simulink model "dsp_audio_player_v1"  (R2020b)
settings: Solver=FixedStepDiscrete  StartTime=0.0  StopTime=Inf  RelTol=1e-3  EnableMultiTasking=on
undefined symbols (not defined in the file or in its folder): A, data, GPTRIP1SEL, GPTRIP2SEL, TZ1, TZ2
libraries: simulink x8, idelinklib_common x3, c280xlib x3, c2837xDlib x2, dspxfrm3 x2, c2000lib x1, c2802xlib x1
settings Model: ExtModeTrigDuration=8  Creator=adria  LastModifiedBy=tyler
settings OptimizationCC: DefaultUnderspecifiedDataType=single  EnhancedBackFolding=on  PassReuseOutputArgsAs=Individual arguments  MaxStackSize=1024  OptimizeBlockOrder=speed  DifferentSizesBufferReuse=on  OptimizationCustomize=off  DenormalBehavior=FlushToZero  EfficientTunableParamExpr=on
settings DebuggingCC: MultiTaskDSMMsg=none  ParameterTunabilityLossMsg=error
settings HardwareCC: ProdBitPerChar=16  ProdBitPerInt=16  ProdBitPerPointer=32  ProdBitPerSizeT=32  ProdBitPerPtrDiffT=32  ProdLargestAtomicInteger=Integer  ProdLargestAtomicFloat=None  ProdWordSize=16  ProdLongLongMode=on  ProdHWDeviceType=Texas Instruments->C2000
settings SFSimCC: MATLABDynamicMemAlloc=off
settings RTWCC: Description=Embedded Coder  SystemTargetFile=ert.tlc  HardwareBoard=TI Delfino F28379D LaunchPad  TemplateMakefile=ert_default_tmf  GenerateReport=on  Toolchain=Texas Instruments Code Composer Studio (C2000)  LaunchReport=on
settings CodeAppCC: ForceParamTrailComments=on  IgnoreCustomStorageClasses=off  OperatorAnnotations=on  SimulinkDataObjDesc=on  SFDataObjDesc=on  InsertBlockDesc=on
settings ERTTargetCC: CodeReplacementLibrary=TI C28x  ExtModeTransport=3  ExtModeStaticAllocSize=10000

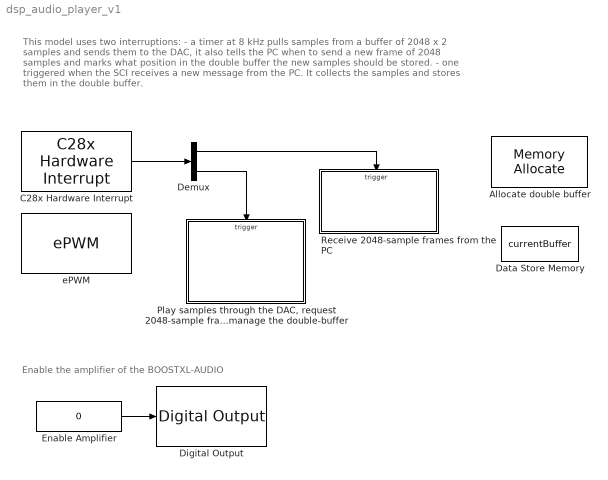
== system dsp_audio_player_v1 ==
  note: This model uses two interruptions:
      | - a timer at 8 kHz pulls samples from a buffer of 2048 x 2 samples and sends them to the DAC, it also tells the PC when to send a new frame of 2048 samples and marks what position in the double buffer the new samples should be stored.
      | - one triggered when the SCI receives a new message from the PC. It collects the samples and stores them in the double buffer.
  note: Enable the amplifier of the BOOSTXL-AUDIO
  Allocate double buffer : idelinklib_common/Memory Allocate  variableName=doubleBuffer  alignThisVariable=off  memoryAlignmentBoundary=4  dataType=uint16  specifyQualifier=off  typeQualifier=volatile  dataDimension=2^12  specifyMemorySection=off  memorySection=mySEC1  bindMemorySection=off  sectionStartAddress=hex2dec('8000')  initializeMemory=on  initialValue=zeros(1,(2^12))
      settings: SourceProductBaseCode=ME
  C28x Hardware Interrupt : c2000lib/Scheduling/C28x Hardware Interrupt  irqnumbers=[9 3]  pienumbers=[1 1]  irqpriorities=[50 30]  irqpreempts=[0 0]  showinput=off  dspchiptype=C280X
      settings: SourceProductName=Embedded Coder Support Package for Texas Instruments C2000 Processors
  Data Store Memory : DataStoreMemory  DataStoreName=currentBuffer  ReadBeforeWriteMsg=warning  WriteAfterWriteMsg=warning  WriteAfterReadMsg=warning  ShowAdditionalParam=off  OutDataTypeStr=uint16
  Demux : Demux  Outputs=2
  Digital Output : c2837xDlib/Digital Output  GPIO_Number=GPIO24~GPIO31  GPIO_Bit0=off  GPIO_BIT0_Toggle=off  GPIO_Bit1=off  GPIO_BIT1_Toggle=off  GPIO_Bit2=on  GPIO_BIT2_Toggle=off  GPIO_Bit3=off  GPIO_BIT3_Toggle=off  GPIO_Bit4=off  GPIO_BIT4_Toggle=off  GPIO_Bit5=off  GPIO_BIT5_Toggle=off  GPIO_Bit6=off  GPIO_BIT6_Toggle=off  GPIO_Bit7=off  GPIO_BIT7_Toggle=off
      settings: SourceProductBaseCode=TIC2000
  Enable Amplifier : Constant  Value=0
  "Play samples through the DAC, request 2048-sample frames from the PC, manage the double-buffer" : Subsystem
  Receive 2048-sample frames from the PC : Subsystem
  ePWM : c2802xlib/ePWM  PwmType=C2000_Type4  useModule=ePWM1  ePWMxLINKTBPRD=Not Linked  periodUnits=Seconds  timerSource=Specify via dialog  timerPeriod_clk=1000  timerPeriod_sec=1/8000  tbshadow=Counter equals to zero  countingMode=Up  phaseActiveEnable=Disable  phaseDirection=Count down after sync  phaseActive=0  synchronizationEnable=off  dcaevt1Sync=off  dcbevt1Sync=off  synchronizationOption=Disable  perSynchronizationOption=Counter equals to period (CTR=PRD)  clockPrescale=1  HSclockPrescale=1  enswap=off  ePWMxAStatus=on  ePWMxAactionLogic1=Do nothing  ePWMxAactionLogic2=Do nothing  ePWMxAactionLogic3=Do nothing  ePWMxAactionLogic4=Set  ePWMxAactionLogic5=Do nothing  ePWMxAactionLogic6=Do nothing  ePWMxACSFenable=off  ePWMxACSFvalue=Forcing disable  ePWMxASFreload=Zero  ePWMxBStatus=off  ePWMxBactionLogic1=Set  ePWMxBactionLogic2=Clear  ePWMxBactionLogic3=Do nothing  ePWMxBactionLogic4=Do nothing  ePWMxBactionLogic5=Clear  ePWMxBactionLogic6=Set  ePWMxBCSFenable=off  ePWMxBCSFvalue=Forcing disable  ePWMxBSFreload=Zero  ePWNxBOutWay=off  ePWMxLINKCMPA=Not Linked  CMPAUnits=Percentages  CMPASource=Specify via dialog  CMPAValue_per=50  CMPAValue_clk=50  enCMPAshadow=Counter equals to zero (CTR=Zero)  ePWMxLINKCMPB=Not Linked  CMPBUnits=Clock cycles  CMPBSource=Specify via dialog  CMPBValue_per=50  CMPBValue_clk=32000  enCMPBshadow=Counter equals to zero (CTR=Zero)  ePWMxLINKCMPC=Not Linked  CMPCUnits=Clock cycles  CMPCSource=Specify via dialog  CMPCValue_per=50  CMPCValue_clk=32000  enCMPCshadow=Counter equals to zero (CTR=Zero)  ePWMxLINKCMPD=Not Linked  CMPDUnits=Clock cycles  CMPDSource=Specify via dialog  CMPDValue_per=50  CMPDValue_clk=32000  enCMPDshadow=Counter equals to zero (CTR=Zero)  enableDBePWMxA=off  enableDBePWMxB=off  enhalfcycle=off  DBpolarity=Active high (AH)  DBedgeDelay=Positive  DBSource_ePWMxA=ePWMxA  DBSource_ePWMxB=ePWMxA  DBPeriodUnits=Clock cycles  DBperiodSource=Specify via dialog  REDperiod=0  FEDperiod=0  REDperiod_sec=0  FEDperiod_sec=0  LoadModeDBRED=Immediate without using shadow  LoadModeDBFED=Immediate without using shadow  adcstartModuleA=off  adcrequestEventA=First event  adcstartEventA=Digital Compare Module A Event 1 start of conversion (DCAEVT1.soc)  adcstartEventA_type2=Digital Compare Module A Event 1 start of conversion (DCAEVT1.soc)  adcstartModuleB=off  adcrequestEventB=First event  adcstartEventB=Counter equals to zero (CTR=Zero)  adcstartEventB_type2=Counter equals to zero (CTR=Zero)  intEn=on  intPrd=First event  intSel=Counter equals to zero (CTR=Zero)  intSel_type2=Counter equals to zero (CTR=Zero)  hrpe=off  enHRPWM=off  HRPWM_LoadMode=Counter equals to period (CTR=PRD)  HRPWM_CTLMode=Duty or Period control mode  HRPWM_EDGMode=Both edge  hrpeb=off  enHRPWMB=off  HRPWM_LoadModeB=Counter equals to zero (CTR=ZERO)  HRPWM_CTLModeB=Duty or Period control mode  HRPWM_EDGModeB=Both edge  enHRDBRED=off  enHRDBFED=off  enSFO=on  enautoconv=on  chopperEnable=off  chopperFrequency=1  chopperFirstwidth=1  chopperDuty=12.5%  tripZonesource=Specify via dialog  tzselOSHT1=off  tzselOSHT2=off  tzselOSHT3=off  tzselOSHDCAEV1=off  tzselOSHDCBEV1=off  tzselCBC1=off  tzselCBC2=off  tzselCBC3=off  tzselCBCDCAEV2=off  tzselCBCDCBEV2=off  tzselOSHT4=off  tzselOSHT5=off  tzselOSHT6=off  tzselCBC4=off  tzselCBC5=off  tzselCBC6=off  enTzOstIntr=off  enTzCbcIntr=off  enTzDCAEVT1Intr=off  enTzDCAEVT2Intr=off  enTzDCBEVT1Intr=off  enTzDCBEVT2Intr=off  ePWMxAforced=No action  ePWMxBforced=No action  DCAEVT1forced=No action  DCBEVT1forced=No action  DCAEVT2forced=No action  DCBEVT2forced=No action  dcah=Trip Zone 1 input (TZ1)  dcal=Trip Zone 2 input (TZ2)  dcbh=Trip Zone 1 input (TZ1)  dcbl=Trip Zone 2 input (TZ2)  dcah_type2=GPTRIP1SEL/(TZ1)  dcal_type2=GPTRIP2SEL/(TZ2)  dcbh_type2=GPTRIP1SEL/(TZ1)  dcbl_type2=GPTRIP2SEL/(TZ2)  gendcaevt1=Event disabled  gendcaevt2=Event disabled  gendcbevt1=Event disabled  gendcbevt2=Event disabled  dcaevt1src=DCAEVT1 with sync  dcaevt2src=DCAEVT2 with sync  dcbevt1src=DCBEVT1 with sync  dcbevt2src=DCBEVT2 with sync  pulsesel=Counter equals to zero (CTR=Zero)  blankinv=off  blankoffset=0  blankwidth=0  evsrcsel=Filtered version of DCAEVT1 (DCAEVT1FILT)  encape=off
      settings: SourceProductName=Embedded Coder Support Package for Texas Instruments C2000 Processors
  wires:
  C28x Hardware Interrupt/1 -> Demux/1
  Demux/1 -> Receive 2048-sample frames from the PC/Trigger
  Demux/2 -> "Play samples through the DAC, request 2048-sample frames from the PC, manage the double-buffer"/Trigger
  Enable Amplifier/1 -> Digital Output/1

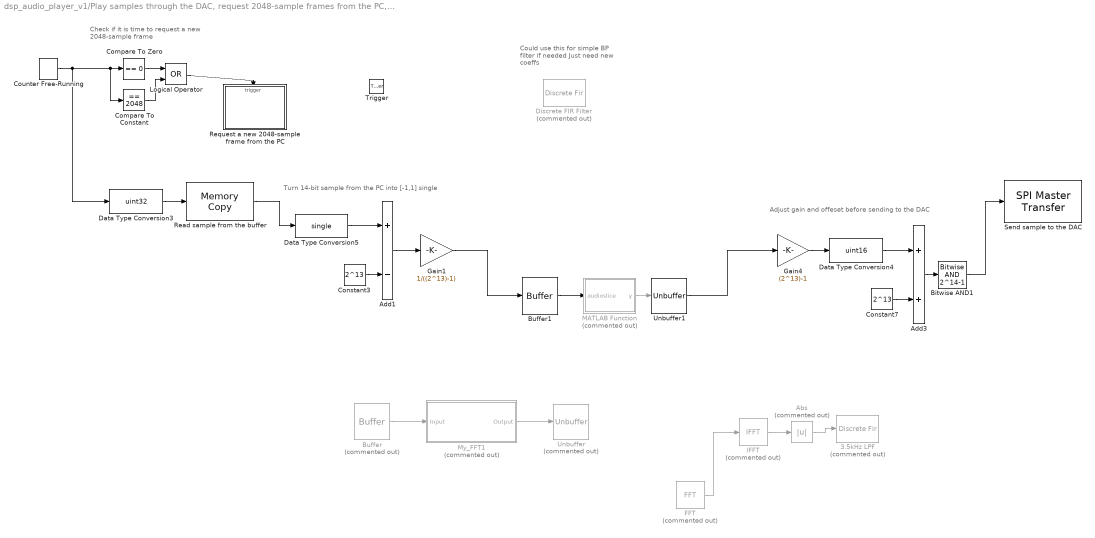
== system dsp_audio_player_v1/Play samples through the DAC, request 2048-sample frames from the PC, manage the double-buffer ==
  note: Could use this for
      | simple BP filter if needed
      | Just need new coeffs
  note: Turn 14-bit sample from the PC into [-1,1] single
  note: Adjust gain and offeset before sending to the DAC
  note: Check if it is time to request
      | a new 2048-sample frame
  Trigger : TriggerPort  TriggerType=function-call  VariantControl=Variant  PortDimensions=1
  3.5kHz LPF : DiscreteFir  Commented=on  Coefficients=[-0.000400517864648427,-0.00597270631126555,-0.00588600875883281,0.00305220673006901,0.00340984153034900,-0.00584791328673356,-0.000942482039609760,0.00831300701616265,-0.00350292218202603,-0.00903364920390202,0.00977259721520285,0.00633489663026340,-0.0164864938688951,0.00112630892188619,0.0210980048311115,-0.0137454614242812,-0.0201583607432012,0.0305294671131217,0.00951594876559339,-0.0490740358099981,0.0166730488518273,0.0660460111384453,-0.0743550579470649,-0.0779651266053814,0.307083541990112,0.582258998534139,0.307083541990112,-0.0779651266053814,-0.0743550579470649,0.0660460111384453,0.0166730488518273,-0.0490740358099981,0.00951594876559339,0.0305294671131217,-0.0201583607432012,-0.0137454614242812,0.0210980048311115,0.00112630892188619,-0.0164864938688951,0.00633489663026340,0.00977259721520285,-0.00903364920390202,-0.00350292218202603,0.00831300701616265,-0.000942482039609760,-0.00584791328673356,0.00340984153034900,0.00305220673006901,-0.00588600875883281,-0.00597270631126555,-0.000400517864648427]
  Abs : Abs  Commented=on
  Add1 : Sum  Inputs=+-
  Add3 : Sum
  Bitwise AND1 : simulink/Logic and Bit Operations/Bitwise Operator  logicop=AND  UseBitMask=on  BitMask=2^14-1  BitMaskRealWorld=Stored Integer
  Buffer : Buffer  Commented=on  N=16  V=15  OutputFrames=off
  Buffer1 : Buffer  N=2048  V=2047  OutputFrames=off
  Compare To Constant : simulink/Logic and Bit Operations/Compare To Constant  relop===  const=2048  OutDataTypeStr=boolean
  Compare To Zero : simulink/Logic and Bit Operations/Compare To Zero  relop===  OutDataTypeStr=boolean
  Constant3 : Constant  Value=2^13  OutDataTypeStr=single
  Constant7 : Constant  Value=2^13  OutDataTypeStr=uint16
  Counter Free-Running : simulink/Sources/Counter Free-Running  NumBits=12  tsamp=-1
  Data Type Conversion3 : DataTypeConversion  OutDataTypeStr=uint32
  Data Type Conversion4 : DataTypeConversion  OutDataTypeStr=uint16
  Data Type Conversion5 : DataTypeConversion  OutDataTypeStr=single
  Discrete FIR Filter : DiscreteFir  Commented=on  Coefficients="[-0.000810102636137497\t-0.000392374131282647\t-4.06563948247084e-05\t0.000767451730429069\t0.00204102792071147\t0.00363434793640914\t0.00522314138161502\t0.00632871351818929\t0.00639886630822526\t0.00494089174170842\t0.00168166719513044\t-0.00327772717740523\t-0.00935730346277267\t-0.0154836748342822\t-0.0201875759335370\t-0.0218139413210731\t-0.0188190039298270\t-0.0101023307256181\t0.00469465139069746\t0.0249940309565858\t0.0492440262935009\t0.0750604816349442\t0.0995424525458068\t0.119710733564489\t0.132986042515205\t0.137615586465308\t0.132986042515205\t0.119710733564489\t0.0995424525458068\t0.0750604816349442\t0.0492440262935009\t0.0249940309565858\t0.00469465139069746\t-0.0101023307256181\t-0.0188190039298270\t-0.0218139413210731\t-0.0201875759335370\t-0.0154836748342822\t-0.00935730346277267\t-0.00327772717740523\t0.00168166719513044\t0.00494089174170842\t0.00639886630822526\t0.00632871351818929\t0.00522314138161502\t0.00363434793640914\t0.00204102792071147\t0.000767451730429069\t-4.06563948247084e-05\t-0.000392374131282647\t-0.000810102636137497]"
  FFT : dspxfrm3/FFT  Commented=on  FFTImplementation=Auto  CompMethod=Table lookup  TableOpt=NEW  TableOptActive=Speed  BitRevOrder=off  Normalize=off  InheritFFTLength=on  FFTLength=64  WrapInput=on  roundingMode=Floor  overflowMode=off  firstCoeffDataTypeStr=Inherit: Same word length as input  firstCoeffLastDataTypeStr=Inherit: Same word length as input  outputMin=[]  outputMax=[]
  Gain1 : Gain  Gain=1/((2^13)-1)
  Gain4 : Gain  Gain=(2^13)-1
  IFFT : dspxfrm3/IFFT  Commented=on  FFTImplementation=Auto  CompMethod=Table lookup  TableOpt=NEW  TableOptActive=Speed  BitRevOrder=off  cs_in=off  Normalize=on  InheritFFTLength=on  FFTLength=64  WrapInput=on  mode=Complex  outSamplingMode=Sample based  roundingMode=Floor  overflowMode=off  firstCoeffDataTypeStr=Inherit: Same word length as input  firstCoeffLastDataTypeStr=Inherit: Same word length as input  outputMin=[]  outputMax=[]
  Logical Operator : Logic  Operator=OR  AllPortsSameDT=off  OutDataTypeStr=boolean
  MATLAB Function : MATLAB Function  Commented=on  TreatAsAtomicUnit=on
  My_FFT1 : Subsystem  Commented=on
  Read sample from the buffer : idelinklib_common/Memory Copy  copyFrom=Specified source code symbol  copyFromAddressSource=Specify via dialog  copyFromAddress=hex2dec('00001000')  copyFromSrcCode=doubleBuffer  dataTypeFrom=uint16  dataDimensionFrom=1  useOffsetFrom=on  offsetFromSrc=Input port  offsetFrom=0  strideFrom=1  copyTo=Output port  copyToAddressSource=Specify via dialog  copyToAddress=hex2dec('00002000')  copyToSrcCode=myVariable  dataTypeTo=uint16  useOffsetTo=off  offsetToSrc=Input port  offsetTo=0  strideTo=1  sampleTime=-1  useInitValue=off  initValueSrc=Specify constant value  initValue=1  initValueSrcCode=myInitValueVariable  useAsMask=off  maskOperator=bitwise AND  useTermValue=off  termValue=1  isRealtimeEnabled=off  emitCCBeforeWrite=off  CCBeforeWrite=/* Custom Code Before Write*/  emitCCAfterWrite=off  CCAfterWrite=/* Custom Code After Write*/  useDMACopy=off  enableBlockingMode=off
      settings: SourceProductBaseCode=ME
  Request a new 2048-sample frame from the PC : Subsystem
  Send sample to the DAC : c280xlib/SPI Master Transfer  SPISelect=SPI_B  ClockPolarity=Rising_edge  ClockPhase=Delay_half_cycle  SPIModule=uint32(0)  Mode=Master  BusSpeed=uint32(1000000)  FirstBitToTransfer=Most significant bit (MSB)  ClockMode=0  BlockFunction=Transfer  EnableRegisterAddress=off  RegisterAddress=0  OutputDataType=int8  OutputDataLength=1  DataBits=16  UseCustomSSPin=Explicit GPIO calls  ActiveLowSSPin=Active low  Pin=27
      settings: SourceProductName=Embedded Coder Support Package for Texas Instruments C2000 Processors
  Unbuffer : Unbuffer  Commented=on
  Unbuffer1 : Unbuffer
  wires:
  Data Type Conversion3/1 -> Read sample from the buffer/1
  Compare To Zero/1 -> Logical Operator/1
  Compare To Constant/1 -> Logical Operator/2
  Logical Operator/1 -> Request a new 2048-sample frame from the PC/Trigger
  Counter Free-Running/1 -> Compare To Constant/1, Compare To Zero/1, Data Type Conversion3/1
  Add3/1 -> Bitwise AND1/1
  Gain4/1 -> Data Type Conversion4/1
  Constant7/1 -> Add3/2
  Data Type Conversion4/1 -> Add3/1
  Constant3/1 -> Add1/2
  Data Type Conversion5/1 -> Add1/1
  Add1/1 -> Gain1/1
  Read sample from the buffer/1 -> Data Type Conversion5/1
  Bitwise AND1/1 -> Send sample to the DAC/1
  My_FFT1/1(Output) -> Unbuffer/1
  Buffer/1 -> My_FFT1/1(Input)
  Gain1/1 -> Buffer1/1
  Abs/1 -> 3.5kHz LPF/1
  FFT/1 -> IFFT/1
  IFFT/1 -> Abs/1
  Buffer1/1 -> MATLAB Function/1(audioslice)
  MATLAB Function/1(y) -> Unbuffer1/1
  Unbuffer1/1 -> Gain4/1

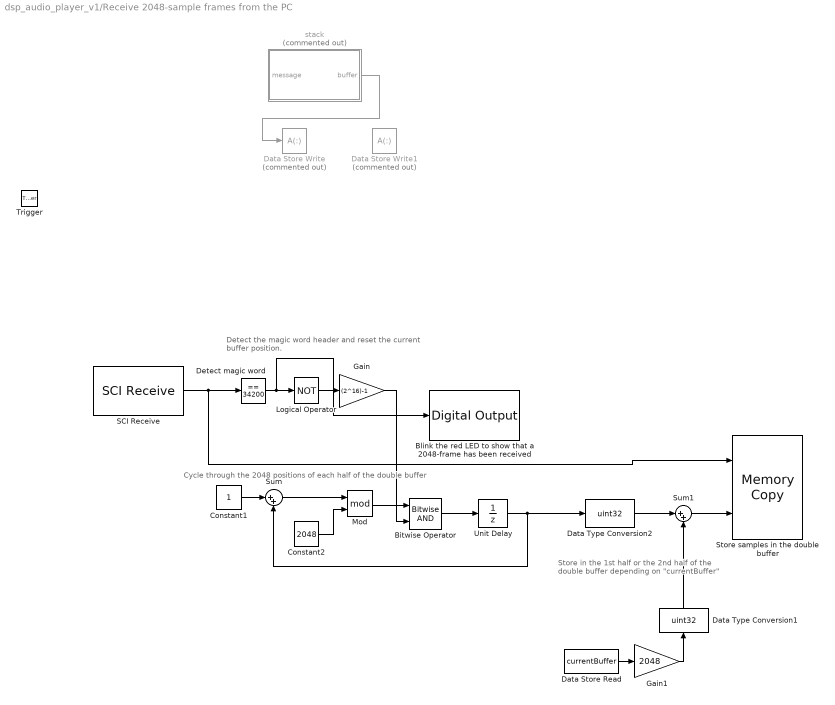
== system dsp_audio_player_v1/Receive 2048-sample frames from the PC ==
  note: Store in the 1st half or the 2nd half
      | of the double buffer depending on
      | "currentBuffer"
  note: Cycle through the 2048 positions of each half of the double buffer
  note: Detect the magic word header and
      | reset the current buffer position.
  Trigger : TriggerPort  TriggerType=function-call  VariantControl=Variant  PortDimensions=1
  Bitwise Operator : simulink/Logic and Bit Operations/Bitwise Operator  logicop=AND  UseBitMask=off  NumInputPorts=2  BitMask=bin2dec('11011001')  BitMaskRealWorld=Stored Integer
  Blink the red LED to show that a 2048-frame has been received : c2837xDlib/Digital Output  GPIO_Number=GPIO32~GPIO39  GPIO_Bit0=off  GPIO_BIT0_Toggle=off  GPIO_Bit1=off  GPIO_BIT1_Toggle=off  GPIO_Bit2=on  GPIO_BIT2_Toggle=on  GPIO_Bit3=off  GPIO_BIT3_Toggle=off  GPIO_Bit4=off  GPIO_BIT4_Toggle=on  GPIO_Bit5=off  GPIO_BIT5_Toggle=off  GPIO_Bit6=off  GPIO_BIT6_Toggle=off  GPIO_Bit7=off  GPIO_BIT7_Toggle=off
      settings: SourceProductBaseCode=TIC2000
  Constant1 : Constant  OutDataTypeStr=uint16  SampleTime=-1
  Constant2 : Constant  Value=2048  OutDataTypeStr=uint16  SampleTime=-1
  Data Store Read : DataStoreRead  DataStoreName=currentBuffer
  Data Store Write : DataStoreWrite  Commented=on  DataStoreElements=A(:)
  Data Store Write1 : DataStoreWrite  Commented=on  DataStoreElements=A(:)
  Data Type Conversion1 : DataTypeConversion  OutDataTypeStr=uint32
  Data Type Conversion2 : DataTypeConversion  OutDataTypeStr=uint32
  Detect magic word : simulink/Logic and Bit Operations/Compare To Constant  relop===  const=34200  OutDataTypeStr=boolean
  Gain : Gain  Gain=(2^16)-1  OutDataTypeStr=uint16
  Gain1 : Gain  Gain=2048  OutDataTypeStr=uint16
  Logical Operator : Logic  Operator=NOT  AllPortsSameDT=off  OutDataTypeStr=boolean
  Mod : Math  Operator=mod  SaturateOnIntegerOverflow=on
  SCI Receive : c280xlib/SCI Receive  sciModule=A  dataHead=''  dataTail=''  dataType=uint16  dataDim=1  initValue=0  errOption=Output the last received value  errValue=0  sampleTime=-1  outputStatus=off  postInterrupt=on  numFifo=2
      settings: SourceProductName=Embedded Coder Support Package for Texas Instruments C2000 Processors
  Store samples in the double buffer : idelinklib_common/Memory Copy  copyFrom=Input port  copyFromAddressSource=Specify via dialog  copyFromAddress=hex2dec('00001000')  copyFromSrcCode=myVariableSrc  dataTypeFrom=uint16  dataDimensionFrom=1  useOffsetFrom=off  offsetFromSrc=Specify via dialog  offsetFrom=0  strideFrom=1  copyTo=Specified source code symbol  copyToAddressSource=Specify via dialog  copyToAddress=hex2dec('00002000')  copyToSrcCode=doubleBuffer  dataTypeTo=uint16  useOffsetTo=on  offsetToSrc=Input port  offsetTo=0  strideTo=1  sampleTime=-1  useInitValue=off  initValueSrc=Specify constant value  initValue=1  initValueSrcCode=myInitValueVariable  useAsMask=off  maskOperator=bitwise AND  useTermValue=off  termValue=1  isRealtimeEnabled=off  emitCCBeforeWrite=off  CCBeforeWrite=/* Custom Code Before Write*/  emitCCAfterWrite=off  CCAfterWrite=/* Custom Code After Write*/  useDMACopy=off  enableBlockingMode=off
      settings: SourceProductBaseCode=ME
  Sum : Sum  Inputs=|++
  Sum1 : Sum  Inputs=|++
  Unit Delay : UnitDelay  SampleTime=-1  HasFrameUpgradeWarning=on
  stack : Subsystem  Commented=on
  wires:
  stack/1(buffer) -> Data Store Write/1
  Unit Delay/1 -> Data Type Conversion2/1, Sum/2
  Detect magic word/1 -> Logical Operator/1, Blink the red LED to show that a 2048-frame has been received/1
  Constant1/1 -> Sum/1
  Sum/1 -> Mod/1
  Constant2/1 -> Mod/2
  SCI Receive/1 -> Detect magic word/1, Store samples in the double buffer/1
  Mod/1 -> Bitwise Operator/1
  Gain/1 -> Bitwise Operator/2
  Bitwise Operator/1 -> Unit Delay/1
  Data Store Read/1 -> Gain1/1
  Data Type Conversion2/1 -> Sum1/1
  Sum1/1 -> Store samples in the double buffer/2
  Gain1/1 -> Data Type Conversion1/1
  Data Type Conversion1/1 -> Sum1/2
  Logical Operator/1 -> Gain/1

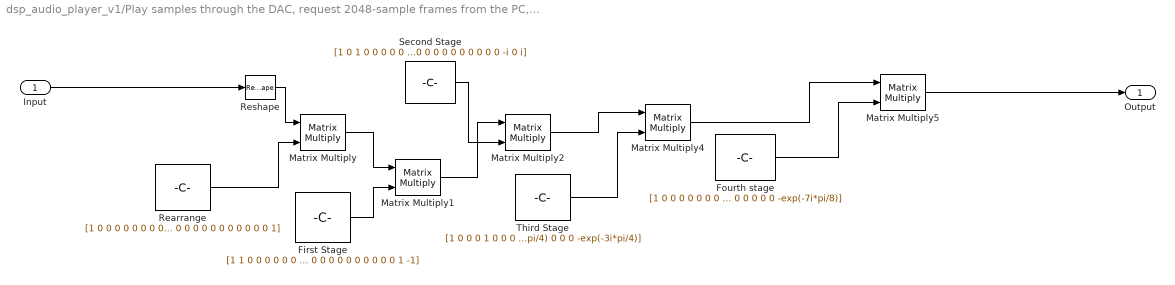
== system dsp_audio_player_v1/Play samples through the DAC, request 2048-sample frames from the PC, manage the double-buffer/My_FFT1 ==
  Input : Inport
  First Stage : Constant  Value=|  VectorParams1D=off  SampleTime=-1
      | [1 1 0 0 0 0 0 0 0 0 0 0 0 0 0 0;
      |  1 -1 0 0 0 0 0 0 0 0 0 0 0 0 0 0;
      |  0 0 1 1 0 0 0 0 0 0 0 0 0 0 0 0;
      |  0 0 1 -1 0 0 0 0 0 0 0 0 0 0 0 0;
      |  0 0 0 0 1 1 0 0 0 0 0 0 0 0 0 0;
      |  0 0 0 0 1 -1 0 0 0 0 0 0 0 0 0 0;
      |  0 0 0 0 0 0 1 1 0 0 0 0 0 0 0 0;
      |  0 0 0 0 0 0 1 -1 0 0 0 0 0 0 0 0;
      |  0 0 0 0 0 0 0 0 1 1 0 0 0 0 0 0;
      |  0 0 0 0 0 0 0 0 1 -1 0 0 0 0 0 0;
      |  0 0 0 0 0 0 0 0 0 0 1 1 0 0 0 0;
      |  0 0 0 0 0 0 0 0 0 0 1 -1 0 0 0 0;
      |  0 0 0 0 0 0 0 0 0 0 0 0 1 1 0 0;
      |  0 0 0 0 0 0 0 0 0 0 0 0 1 -1 0 0;
      |  0 0 0 0 0 0 0 0 0 0 0 0 0 0 1 1;
      |  0 0 0 0 0 0 0 0 0 0 0 0 0 0 1 -1]
  Fourth stage : Constant  Value=|  VectorParams1D=off  SampleTime=-1
      | [1 0 0 0 0 0 0 0 1 0 0 0 0 0 0 0;
      |  0 1 0 0 0 0 0 0 0 1 0 0 0 0 0 0;
      |  0 0 1 0 0 0 0 0 0 0 1 0 0 0 0 0;
      |  0 0 0 1 0 0 0 0 0 0 0 1 0 0 0 0;
      |  0 0 0 0 1 0 0 0 0 0 0 0 1 0 0 0;
      |  0 0 0 0 0 1 0 0 0 0 0 0 0 1 0 0;
      |  0 0 0 0 0 0 1 0 0 0 0 0 0 0 1 0;
      |  0 0 0 0 0 0 0 1 0 0 0 0 0 0 0 1;
      |  1 0 0 0 0 0 0 0 -1 0 0 0 0 0 0 0;
      |  0 exp(-1i*pi/8) 0 0 0 0 0 0 0 -exp(-1i*pi/8) 0 0 0 0 0 0;
      |  0 0 exp(-2i*pi/8) 0 0 0 0 0 0 0 -exp(-2i*pi/8) 0 0 0 0 0;
      |  0 0 0 exp(-3i*pi/8) 0 0 0 0 0 0 0 -exp(-3i*pi/8) 0 0 0 0;
      |  0 0 0 0 exp(-4i*pi/8) 0 0 0 0 0 0 0 -exp(-4i*pi/8) 0 0 0;
      |  0 0 0 0 0 exp(-5i*pi/8) 0 0 0 0 0 0 0 -exp(-5i*pi/8) 0 0;
      |  0 0 0 0 0 0 exp(-6i*pi/8) 0 0 0 0 0 0 0 -exp(-6i*pi/8) 0;
      |  0 0 0 0 0 0 0 exp(-7i*pi/8) 0 0 0 0 0 0 0 -exp(-7i*pi/8)]
  Matrix Multiply{,1..2,4..5} (5 alike) : Product  Multiplication=Matrix(*)
  Rearrange : Constant  Value=|  VectorParams1D=off  SampleTime=-1
      | [1 0 0 0 0 0 0 0 0 0 0 0 0 0 0 0;
      |  0 0 0 0 0 0 0 0 1 0 0 0 0 0 0 0;
      |  0 0 0 0 1 0 0 0 0 0 0 0 0 0 0 0;
      |  0 0 0 0 0 0 0 0 0 0 0 0 1 0 0 0;
      |  0 0 1 0 0 0 0 0 0 0 0 0 0 0 0 0;
      |  0 0 0 0 0 0 0 0 0 0 1 0 0 0 0 0;
      |  0 0 0 0 0 0 1 0 0 0 0 0 0 0 0 0;
      |  0 0 0 0 0 0 0 0 0 0 0 0 0 0 1 0;
      |  0 1 0 0 0 0 0 0 0 0 0 0 0 0 0 0;
      |  0 0 0 0 0 0 0 0 0 1 0 0 0 0 0 0;
      |  0 0 0 0 0 1 0 0 0 0 0 0 0 0 0 0;
      |  0 0 0 0 0 0 0 0 0 0 0 0 0 1 0 0;
      |  0 0 0 1 0 0 0 0 0 0 0 0 0 0 0 0;
      |  0 0 0 0 0 0 0 0 0 0 0 1 0 0 0 0;
      |  0 0 0 0 0 0 0 1 0 0 0 0 0 0 0 0;
      |  0 0 0 0 0 0 0 0 0 0 0 0 0 0 0 1]
  Reshape : Reshape  OutputDimensionality=Row vector (2-D)
  Second Stage : Constant  Value=|  VectorParams1D=off  SampleTime=-1
      | [1 0 1 0 0 0 0 0 0 0 0 0 0 0 0 0;
      |  0 1 0 1 0 0 0 0 0 0 0 0 0 0 0 0;
      |  1 0 -1 0 0 0 0 0 0 0 0 0 0 0 0 0;
      |  0 -i 0 i 0 0 0 0 0 0 0 0 0 0 0 0;
      |  0 0 0 0 1 0 1 0 0 0 0 0 0 0 0 0;
      |  0 0 0 0 0 1 0 1 0 0 0 0 0 0 0 0;
      |  0 0 0 0 1 0 -1 0 0 0 0 0 0 0 0 0;
      |  0 0 0 0 0 -i 0 i 0 0 0 0 0 0 0 0;
      |  0 0 0 0 0 0 0 0 1 0 1 0 0 0 0 0;
      |  0 0 0 0 0 0 0 0 0 1 0 1 0 0 0 0;
      |  0 0 0 0 0 0 0 0 1 0 -1 0 0 0 0 0;
      |  0 0 0 0 0 0 0 0 0 -i 0 i 0 0 0 0;
      |  0 0 0 0 0 0 0 0 0 0 0 0 1 0 1 0;
      |  0 0 0 0 0 0 0 0 0 0 0 0 0 1 0 1;
      |  0 0 0 0 0 0 0 0 0 0 0 0 1 0 -1 0;
      |  0 0 0 0 0 0 0 0 0 0 0 0 0 -i 0 i]
  Third Stage : Constant  Value=|  VectorParams1D=off  SampleTime=-1
      | [1 0 0 0 1 0 0 0 0 0 0 0 0 0 0 0;
      |  0 1 0 0 0 1 0 0 0 0 0 0 0 0 0 0;
      |  0 0 1 0 0 0 1 0 0 0 0 0 0 0 0 0;
      |  0 0 0 1 0 0 0 1 0 0 0 0 0 0 0 0;
      |  1 0 0 0 -1 0 0 0 0 0 0 0 0 0 0 0;
      |  0 exp(-i*pi/4) 0 0 0 -exp(-i*pi/4) 0 0 0 0 0 0 0 0 0 0;
      |  0 0 -i 0 0 0 i 0 0 0 0 0 0 0 0 0;
      |  0 0 0 exp(-3i*pi/4) 0 0 0 -exp(-3i*pi/4) 0 0 0 0 0 0 0 0;
      |  0 0 0 0 0 0 0 0 1 0 0 0 1 0 0 0;
      |  0 0 0 0 0 0 0 0 0 1 0 0 0 1 0 0;
      |  0 0 0 0 0 0 0 0 0 0 1 0 0 0 1 0;
      |  0 0 0 0 0 0 0 0 0 0 0 1 0 0 0 1;
      |  0 0 0 0 0 0 0 0 1 0 0 0 -1 0 0 0;
      |  0 0 0 0 0 0 0 0 0 exp(-i*pi/4) 0 0 0 -exp(-i*pi/4) 0 0;
      |  0 0 0 0 0 0 0 0 0 0 -i 0 0 0 i 0;
      |  0 0 0 0 0 0 0 0 0 0 0 exp(-3i*pi/4) 0 0 0 -exp(-3i*pi/4)]
  Output : Outport
  wires:
  Second Stage/1 -> Matrix Multiply2/2
  Matrix Multiply1/1 -> Matrix Multiply2/1
  Matrix Multiply4/1 -> Matrix Multiply5/1
  Fourth stage/1 -> Matrix Multiply5/2
  Third Stage/1 -> Matrix Multiply4/2
  Reshape/1 -> Matrix Multiply/1
  First Stage/1 -> Matrix Multiply1/2
  Matrix Multiply2/1 -> Matrix Multiply4/1
  Matrix Multiply/1 -> Matrix Multiply1/1
  Rearrange/1 -> Matrix Multiply/2
  Input/1 -> Reshape/1
  Matrix Multiply5/1 -> Output/1

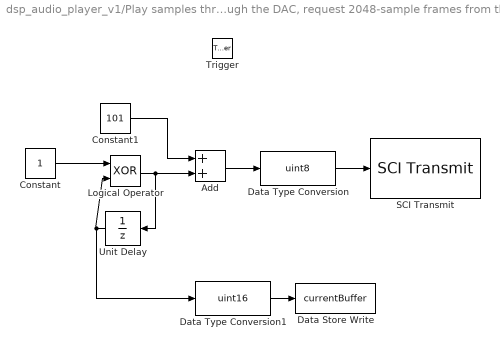
== system dsp_audio_player_v1/Play samples through the DAC, request 2048-sample frames from the PC, manage the double-buffer/Request a new 2048-sample frame from the PC ==
  Trigger : TriggerPort  VariantControl=Variant  PortDimensions=1
  Add : Sum
  Constant : Constant  OutDataTypeStr=boolean  SampleTime=-1
  Constant1 : Constant  Value=101  OutDataTypeStr=uint8  SampleTime=-1
  Data Store Write : DataStoreWrite  DataStoreName=currentBuffer
  Data Type Conversion : DataTypeConversion  OutDataTypeStr=uint8
  Data Type Conversion1 : DataTypeConversion  OutDataTypeStr=uint16
  Logical Operator : Logic  Operator=XOR  AllPortsSameDT=off  OutDataTypeStr=boolean
  SCI Transmit : c280xlib/SCI Transmit  sciModule=A  dataHead=''  dataTail=''  postInterrupt=off  numFifo=1
      settings: SourceProductName=Embedded Coder Support Package for Texas Instruments C2000 Processors
  Unit Delay : UnitDelay  SampleTime=-1  HasFrameUpgradeWarning=on
  wires:
  Constant1/1 -> Add/1
  Unit Delay/1 -> Data Type Conversion1/1, Logical Operator/2
  Constant/1 -> Logical Operator/1
  Add/1 -> Data Type Conversion/1
  Logical Operator/1 -> Add/2, Unit Delay/1
  Data Type Conversion/1 -> SCI Transmit/1
  Data Type Conversion1/1 -> Data Store Write/1

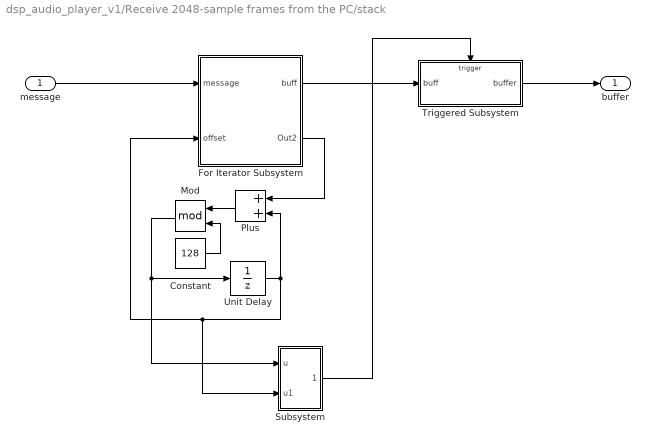
== system dsp_audio_player_v1/Receive 2048-sample frames from the PC/stack ==
  message : Inport
  Constant : Constant  Value=128  SampleTime=-1
  For Iterator Subsystem : Subsystem  TreatAsAtomicUnit=on
  Mod : Math  Operator=mod  SaturateOnIntegerOverflow=on
  Plus : Sum
  Subsystem : Subsystem
  Triggered Subsystem : Subsystem  TreatAsAtomicUnit=on
  Unit Delay : UnitDelay  InitialCondition=127  SampleTime=-1  HasFrameUpgradeWarning=on
  buffer : Outport
  wires:
  Triggered Subsystem/1(buffer) -> buffer/1
  Mod/1 -> Subsystem/1(u), Unit Delay/1
  message/1 -> For Iterator Subsystem/1(message)
  Plus/1 -> Mod/1
  Unit Delay/1 -> Plus/2, Subsystem/2(u1), For Iterator Subsystem/2(offset)
  For Iterator Subsystem/2(Out2) -> Plus/1
  Constant/1 -> Mod/2
  For Iterator Subsystem/1(buff) -> Triggered Subsystem/1(buff)
  Subsystem/1(Out1) -> Triggered Subsystem/Trigger

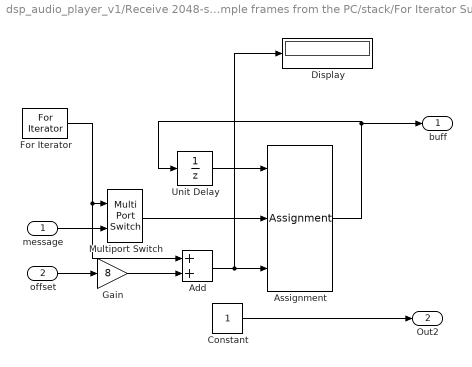
== system dsp_audio_player_v1/Receive 2048-sample frames from the PC/stack/For Iterator Subsystem ==
  message : Inport
  offset : Inport  Port=2
  Add : Sum
  Assignment : Assignment  DiagnosticForDimensions=Warning  IndexOptions=Index vector (port)  Indices=1  OutputSizes=1
  Constant : Constant  SampleTime=-1
  Display : Display
  For Iterator : ForIterator  IterationLimit=8
  Gain : Gain  Gain=8
  Multiport Switch : MultiPortSwitch  Inputs=1
  Unit Delay : UnitDelay  InitialCondition=zeros(8*128,1)  SampleTime=-1  HasFrameUpgradeWarning=on
  buff : Outport
  Out2 : Outport  Port=2
  wires:
  Unit Delay/1 -> Assignment/1
  Assignment/1 -> Unit Delay/1, buff/1
  message/1 -> Multiport Switch/2
  For Iterator/1 -> Add/1, Multiport Switch/1
  Multiport Switch/1 -> Assignment/2
  Add/1 -> Display/1, Assignment/3
  offset/1 -> Gain/1
  Constant/1 -> Out2/1
  Gain/1 -> Add/2

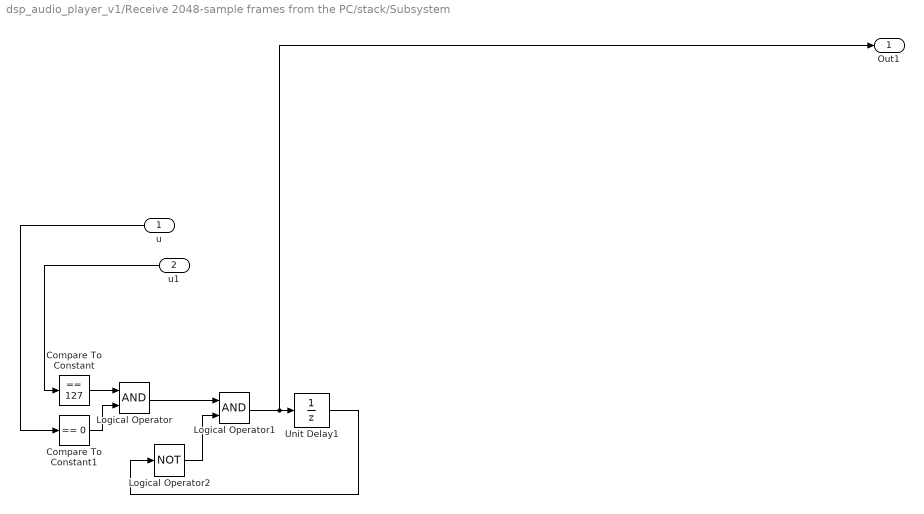
== system dsp_audio_player_v1/Receive 2048-sample frames from the PC/stack/Subsystem ==
  u : Inport
  u1 : Inport  Port=2
  Compare To Constant : simulink/Logic and Bit Operations/Compare To Constant  relop===  const=127  OutDataTypeStr=boolean
  Compare To Constant1 : simulink/Logic and Bit Operations/Compare To Constant  relop===  const=0  OutDataTypeStr=boolean
  Logical Operator : Logic  AllPortsSameDT=off  OutDataTypeStr=boolean
  Logical Operator1 : Logic  AllPortsSameDT=off  OutDataTypeStr=boolean
  Logical Operator2 : Logic  Operator=NOT  AllPortsSameDT=off  OutDataTypeStr=boolean
  Unit Delay1 : UnitDelay  InitialCondition=127  SampleTime=-1  HasFrameUpgradeWarning=on
  Out1 : Outport
  wires:
  Compare To Constant1/1 -> Logical Operator/2
  u1/1 -> Compare To Constant/1
  Unit Delay1/1 -> Logical Operator2/1
  Logical Operator/1 -> Logical Operator1/1
  Logical Operator1/1 -> Out1/1, Unit Delay1/1
  Logical Operator2/1 -> Logical Operator1/2
  u/1 -> Compare To Constant1/1
  Compare To Constant/1 -> Logical Operator/1

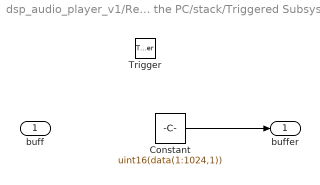
== system dsp_audio_player_v1/Receive 2048-sample frames from the PC/stack/Triggered Subsystem ==
  buff : Inport
  Trigger : TriggerPort  VariantControl=Variant
  Constant : Constant  Value=uint16(data(1:1024,1))  SampleTime=-1
  buffer : Outport
  wires:
  Constant/1 -> buffer/1

== matlab function dsp_audio_player_v1/Play samples through the DAC, request 2048-sample frames from the PC, manage the double-buffer/MATLAB Function ==
  data: audioslice input; y output
function y = fcn(audioslice)
win = sqrt(hann(1024,"periodic"));
overlapLength = floor(numel(win)/2);
fftLength = 2^nextpow2(numel(win) + 1);
ystft = stft(audioslice, ...
        "Window",win, ...
        "OverlapLength",overlapLength, ...
        "FFTLength",fftLength, ...
        "Centered",true);
y = istft(ystft, ...
    "Window",win, ...
    "OverlapLength",overlapLength, ...
    "FFTLength",fftLength, ...
    "ConjugateSymmetric",true);
